simulink model "contrast_stretch_color"  (R2022a)
settings: Solver=FixedStepDiscrete  StartTime=0.0  StopTime=Ts_240p*20  RelTol=1e-3
InitFcn:
  | Ts = 1e-3;
  | Ts_240p = 402*324*Ts;
  | Ts_480p = 525*800*Ts;
undefined symbols (not defined in the file or in its folder): gray, Rec, SDTV
libraries: hdlsllib x8, visionhdlconversions x2, visionhdlio x2, visionconversions x1, visionanalysis x1, dspvision x1
settings Model: DataTypeOverride=Off  ModifiedByFormat=The MathWorks Inc.  NumberOfSteps=10  Creator=The MathWorks, Inc.  LastModifiedBy=The MathWorks Inc.
settings SolverCC: AlgebraicLoopSolver=TrustRegion
settings DataIOCC: LimitDataPoints=on  SaveFormat=Array  SaveOutput=off  SaveTime=off  ReturnWorkspaceOutputs=off
settings OptimizationCC: BlockReduction=off  ConditionallyExecuteInputs=off  DefaultParameterBehavior=Inlined  LifeSpan=inf
settings DebuggingCC: AlgebraicLoopMsg=error  SolverPrmCheckMsg=warning  SingleTaskRateTransMsg=error  ParameterPrecisionLossMsg=none  UnconnectedInputMsg=warning  UnconnectedOutputMsg=warning  UnconnectedLineMsg=warning  AllowSymbolicDim=off  SFUnexpectedBacktrackingDiag=warning  SFNoUnconditionalDefaultTransitionDiag=warning  SFExecutionAtInitializationDiag=none  SFMachineParentedDataDiag=warning  IntegerSaturationMsg=none  ArithmeticOperatorsInVariantConditions=warning
settings HardwareCC: ProdBitPerPointer=32  ProdBitPerSizeT=32  ProdBitPerPtrDiffT=32  ProdLargestAtomicFloat=None  ProdIntDivRoundTo=Undefined  ProdEndianess=Unspecified  ProdWordSize=32  ProdHWDeviceType=ASIC/FPGA->ASIC/FPGA  ProdEqTarget=off
settings ModelReferenceCC: PropagateSignalLabelsOutOfModel=off
settings SFSimCC: SimUseLocalCustomCode=off  CustomCodeUndefinedFunction=UseInterfaceOnly
settings RTWCC: RTWUseLocalCustomCode=off  DLArmComputeVersion=19.05
settings CodeAppCC: StateflowObjectComments=on
settings GRTTargetCC: TargetLangStandard=C89/C90 (ANSI)
settings ConfigComp: CovMetricSettings=dw  CovSaveCumulativeToWorkspaceVar=on  CovSaveSingleToWorkspaceVar=on  CovExternalEMLEnable=off  CovSFcnEnable=off

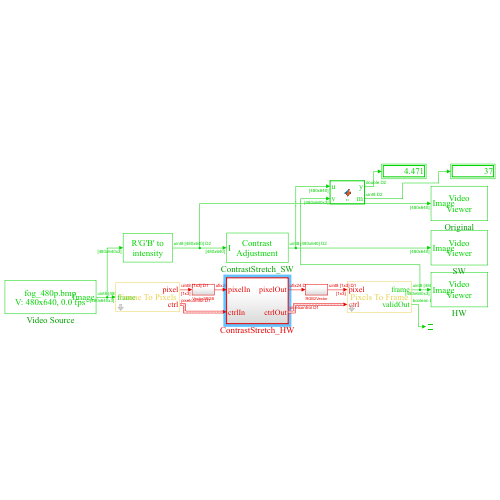
[thumbnail: Simulink's stored preview of the top-level diagram]
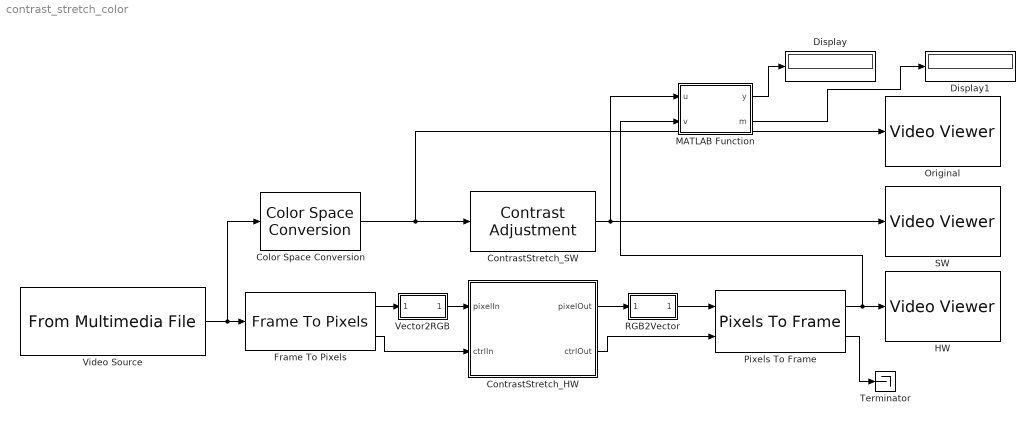
== system contrast_stretch_color ==
  Color Space Conversion : visionconversions/Color Space  Conversion  conversion=Obsolete  conversionActive=R'G'B' to intensity  wp_str=D65  rec=Rec. 601 (SDTV)  sys=1125/60/2:1  imagePorts=One multidimensional signal
  ContrastStretch_HW : Subsystem  TreatAsAtomicUnit=on
  ContrastStretch_SW : visionanalysis/Contrast Adjustment  methodInputRange=Range determined by saturating outlier pixels  rangeIn=[0 73]  fracSaturate=[0.15 0.15]  isBinNum=on  binNum=256  methodOutputRange=Full data type range  rangeOut=[0 255]  roundingMode=Floor  overflowMode=off  prod1Mode=Binary point scaling  prod1WordLength=32  prod1FracLength=16  prod2Mode=Binary point scaling  prod2WordLength=32  prod2FracLength=16
      settings: SourceProductBaseCode=VP
  Display : Display
  Display1 : Display
  Frame To Pixels : visionhdlio/Frame To Pixels  NumComponents=3  NumPixels=1  VideoFormat=480p  ActivePixelsPerLine=640  ActiveVideoLines=480  TotalPixelsPerLine=800  TotalVideoLines=525  StartingActiveLine=36  FrontPorch=16  SampleTime=0  VideoFormatCache=480p  ActivePixelsPerLineCache=32  ActiveVideoLinesCache=18  TotalPixelsPerLineCache=42  TotalVideoLinesCache=28  StartingActiveLineCache=6  FrontPorchCache=5
      settings: SourceProductBaseCode=VT
  HW : VideoViewer  colormapValue=gray(256)  FigPos=[522 705 688 515]
  MATLAB Function : MATLAB Function  TreatAsAtomicUnit=on
  Original : VideoViewer  colormapValue=gray(256)  FigPos=[870 897 688 510]
  Pixels To Frame : visionhdlio/Pixels To Frame  NumComponents=3  NumPixels=1  VideoFormat=480p  ActivePixelsPerLine=640  ActiveVideoLines=480  TotalPixelsPerLine=800  TotalVideoLines=525  VideoFormatCache=480p  ActivePixelsPerLineCache=32  ActiveVideoLinesCache=18  TotalPixelsPerLineCache=42  TotalVideoLinesCache=28
      settings: SourceProductBaseCode=VT
  RGB2Vector : Subsystem
  SW : VideoViewer  colormapValue=gray(256)  FigPos=[295 870 688 514]
  Terminator : Terminator
  Vector2RGB : Subsystem
  Video Source : dspvision/From Multimedia File  inputFilename=D:\datasets\test_images\fog_480p.bmp  readRange=[1 Inf]  loop=on  numPlays=inf  outputStreams=Video only  videoDataType=uint8  audioDataType=int16  inheritSampleTime=off  userDefinedSampleTime=Ts_480p  noAudioOutput=off  isIntensityVideo=off  fourcc=RGB  colorVideoFormat=One multidimensional signal  outputEOF=off  dataOrg=Column-major  audioFrameSize=1024  computeAudioFrameSize=off  outSamplingMode=Sample based
  wires:
  Pixels To Frame/2 -> Terminator/1
  Pixels To Frame/1 -> MATLAB Function/2(v), HW/1
  Vector2RGB/1(RGB) -> ContrastStretch_HW/1(pixelIn)
  ContrastStretch_HW/1(pixelOut) -> RGB2Vector/1(RGB)
  Video Source/1 -> Frame To Pixels/1, Color Space Conversion/1
  Frame To Pixels/2 -> ContrastStretch_HW/2(ctrlIn)
  Frame To Pixels/1 -> Vector2RGB/1(RGBVector)
  RGB2Vector/1(RGBVector) -> Pixels To Frame/1
  ContrastStretch_HW/2(ctrlOut) -> Pixels To Frame/2
  ContrastStretch_SW/1 -> MATLAB Function/1(u), SW/1
  Color Space Conversion/1 -> ContrastStretch_SW/1, Original/1
  MATLAB Function/1(y) -> Display/1
  MATLAB Function/2(m) -> Display1/1

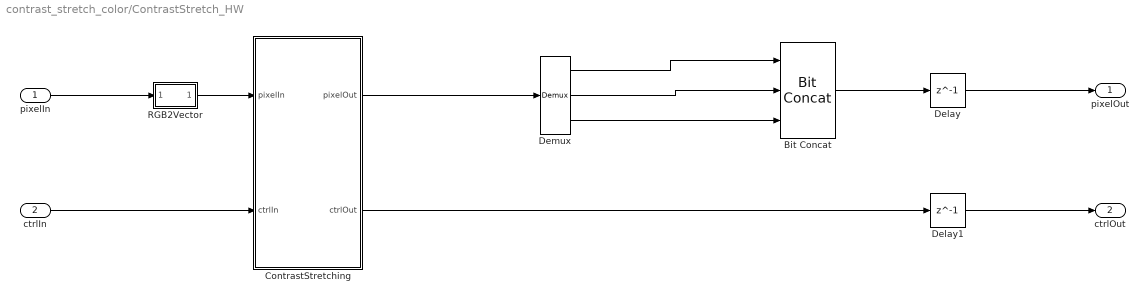
== system contrast_stretch_color/ContrastStretch_HW ==
  pixelIn : Inport
  ctrlIn : Inport  Port=2
  Bit Concat : hdlsllib/Logic and Bit Operations/Bit Concat  numInputs=3
  ContrastStretching : Subsystem  TreatAsAtomicUnit=on
  Delay : Delay  DelayLength=1  InitialCondition=0
  Delay1 : Delay  DelayLength=1  InitialCondition=0
  Demux : Demux  Outputs=3
  RGB2Vector : Subsystem
  pixelOut : Outport  VectorParamsAs1DForOutWhenUnconnected=off
  ctrlOut : Outport  Port=2  VectorParamsAs1DForOutWhenUnconnected=off
  wires:
  ctrlIn/1 -> ContrastStretching/2(ctrlIn)
  pixelIn/1 -> RGB2Vector/1(RGB)
  RGB2Vector/1(RGBVector) -> ContrastStretching/1(pixelIn)
  Bit Concat/1 -> Delay/1
  ContrastStretching/2(ctrlOut) -> Delay1/1
  ContrastStretching/1(pixelOut) -> Demux/1
  Demux/1 -> Bit Concat/1
  Demux/2 -> Bit Concat/2
  Demux/3 -> Bit Concat/3
  Delay/1 -> pixelOut/1
  Delay1/1 -> ctrlOut/1

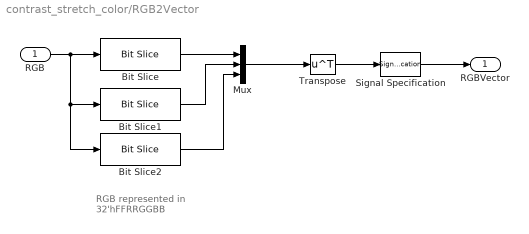
== system contrast_stretch_color/RGB2Vector ==
  note: RGB represented in
      | 32'hFFRRGGBB
  RGB : Inport
  Bit Slice : hdlsllib/Logic and Bit Operations/Bit Slice  lidx=23  ridx=16
      settings: SourceProductBaseCode=SL
  Bit Slice1 : hdlsllib/Logic and Bit Operations/Bit Slice  lidx=15  ridx=8
      settings: SourceProductBaseCode=SL
  Bit Slice2 : hdlsllib/Logic and Bit Operations/Bit Slice  lidx=7  ridx=0
      settings: SourceProductBaseCode=SL
  Mux : Mux  Inputs=3
  Signal Specification : SignalSpecification
  Transpose : Math  Operator=transpose  SignedPower=on
  RGBVector : Outport  VectorParamsAs1DForOutWhenUnconnected=off
  wires:
  Mux/1 -> Transpose/1
  Bit Slice/1 -> Mux/1
  Bit Slice2/1 -> Mux/3
  Bit Slice1/1 -> Mux/2
  RGB/1 -> Bit Slice2/1, Bit Slice1/1, Bit Slice/1
  Transpose/1 -> Signal Specification/1
  Signal Specification/1 -> RGBVector/1

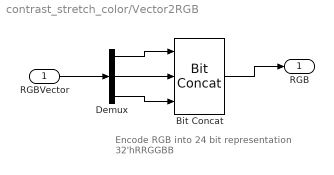
== system contrast_stretch_color/Vector2RGB ==
  note: Encode RGB into 24 bit representation
      | 32'hRRGGBB
  RGBVector : Inport
  Bit Concat : hdlsllib/Logic and Bit Operations/Bit Concat  numInputs=3
  Demux : Demux  Outputs=3
  RGB : Outport  VectorParamsAs1DForOutWhenUnconnected=off
  wires:
  Bit Concat/1 -> RGB/1
  RGBVector/1 -> Demux/1
  Demux/1 -> Bit Concat/1
  Demux/2 -> Bit Concat/2
  Demux/3 -> Bit Concat/3

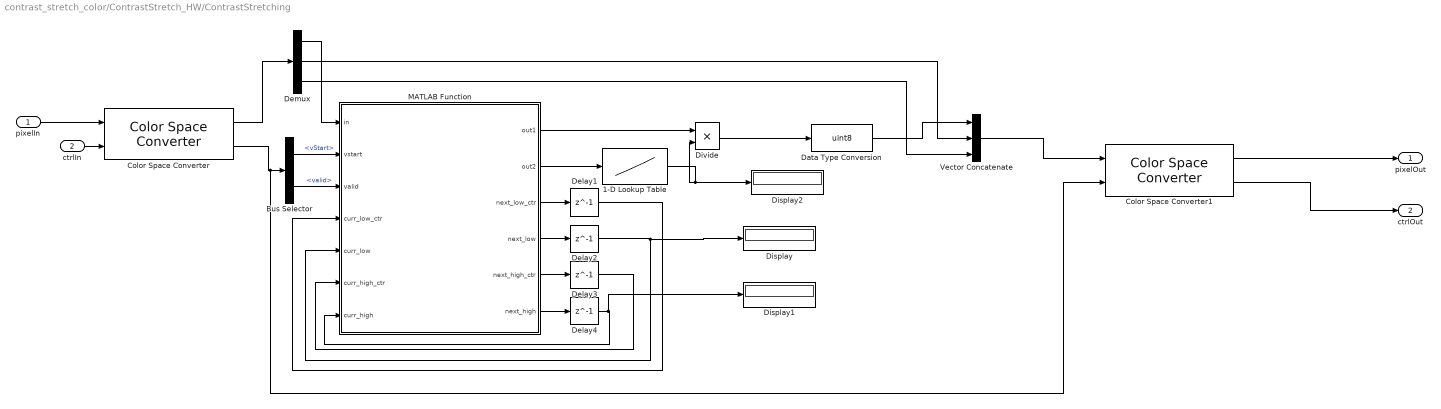
== system contrast_stretch_color/ContrastStretch_HW/ContrastStretching ==
  pixelIn : Inport
  ctrlIn : Inport  Port=2
  1-D Lookup Table : Lookup_n-D  NumberOfTableDimensions=1  LookupTableObject=''  BreakpointsForDimension1=[1:255]  BreakpointsForDimension1FirstPoint=10  BreakpointsForDimension2FirstPoint=10  BreakpointsForDimension1Spacing=12  BreakpointsForDimension2Spacing=12  IndexSearchMethod=Evenly spaced points  Table=1./[1:255]  TableDataTypeStr=fixdt(1,16,15)  InterpMethod=Flat  DiagnosticForOutOfRangeInput=Error  InternalRulePriority=Speed  OutDataTypeStr=fixdt(1,16,15)  RndMeth=Simplest
  Bus Selector : BusSelector  OutputSignals=vStart,valid
  Color Space Converter : visionhdlconversions/Color Space Converter  Conversion=RGB to YCbCr  ConversionStandard=Rec. 601 (SDTV)  ScanningStandard=1250/50/2:1  SimulateUsing=Code generation
      settings: SourceProductBaseCode=VT
  Color Space Converter1 : visionhdlconversions/Color Space Converter  Conversion=YCbCr to RGB  ConversionStandard=Rec. 601 (SDTV)  ScanningStandard=1250/50/2:1  SimulateUsing=Code generation
      settings: SourceProductBaseCode=VT
  Data Type Conversion : DataTypeConversion  OutDataTypeStr=uint8  RndMeth=Floor
  Delay1 : Delay  DelayLength=1  InitialCondition=0
  Delay2 : Delay  DelayLength=1  InitialCondition=100
  Delay3 : Delay  DelayLength=1  InitialCondition=0
  Delay4 : Delay  DelayLength=1  InitialCondition=132
  Demux : Demux  Outputs=3
  Display : Display
  Display1 : Display
  Display2 : Display
  Divide : Product  Inputs=**  RndMeth=Zero
  MATLAB Function : MATLAB Function  TreatAsAtomicUnit=on
  Vector Concatenate : Concatenate  NumInputs=3  Mode=Multidimensional array  ConcatenateDimension=2
  pixelOut : Outport  VectorParamsAs1DForOutWhenUnconnected=off
  ctrlOut : Outport  Port=2  VectorParamsAs1DForOutWhenUnconnected=off
  wires:
  pixelIn/1 -> Color Space Converter/1
  ctrlIn/1 -> Color Space Converter/2
  Color Space Converter/2 -> Color Space Converter1/2, Bus Selector/1
  MATLAB Function/3(next_low_ctr) -> Delay1/1
  Delay1/1 -> MATLAB Function/4(curr_low_ctr)
  MATLAB Function/4(next_low) -> Delay2/1
  Delay2/1 -> Display/1, MATLAB Function/5(curr_low)
  Bus Selector/1 -> MATLAB Function/2(vstart)  "<vStart>"
  Bus Selector/2 -> MATLAB Function/3(valid)  "<valid>"
  MATLAB Function/5(next_high_ctr) -> Delay3/1
  MATLAB Function/6(next_high) -> Delay4/1
  Delay4/1 -> Display1/1, MATLAB Function/7(curr_high)
  Delay3/1 -> MATLAB Function/6(curr_high_ctr)
  MATLAB Function/2(out2) -> 1-D Lookup Table/1
  MATLAB Function/1(out1) -> Divide/1
  1-D Lookup Table/1 -> Display2/1, Divide/2
  Data Type Conversion/1 -> Vector Concatenate/1
  Divide/1 -> Data Type Conversion/1
  Color Space Converter/1 -> Demux/1
  Demux/1 -> MATLAB Function/1(in)
  Demux/3 -> Vector Concatenate/3
  Vector Concatenate/1 -> Color Space Converter1/1
  Color Space Converter1/1 -> pixelOut/1
  Color Space Converter1/2 -> ctrlOut/1
  Demux/2 -> Vector Concatenate/2

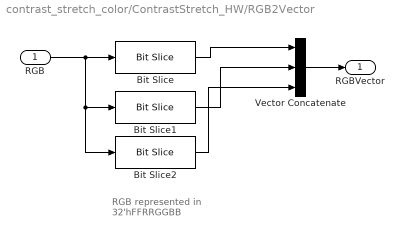
== system contrast_stretch_color/ContrastStretch_HW/RGB2Vector ==
  note: RGB represented in
      | 32'hFFRRGGBB
  RGB : Inport
  Bit Slice : hdlsllib/Logic and Bit Operations/Bit Slice  lidx=23  ridx=16
      settings: SourceProductBaseCode=SL
  Bit Slice1 : hdlsllib/Logic and Bit Operations/Bit Slice  lidx=15  ridx=8
      settings: SourceProductBaseCode=SL
  Bit Slice2 : hdlsllib/Logic and Bit Operations/Bit Slice  lidx=7  ridx=0
      settings: SourceProductBaseCode=SL
  Vector Concatenate : Concatenate  NumInputs=3  Mode=Multidimensional array  ConcatenateDimension=2
  RGBVector : Outport  VectorParamsAs1DForOutWhenUnconnected=off
  wires:
  Bit Slice/1 -> Vector Concatenate/1
  Bit Slice2/1 -> Vector Concatenate/3
  Bit Slice1/1 -> Vector Concatenate/2
  RGB/1 -> Bit Slice2/1, Bit Slice1/1, Bit Slice/1
  Vector Concatenate/1 -> RGBVector/1

== matlab function contrast_stretch_color/MATLAB Function ==
  data: u input; y output; v input; m output
function [y,m] = fcn(u,v)
v = v(:,:,1);
s = size(v);
y = sum(sum(abs(u-v)))/(s(1)*s(2));
m = max(max(abs(u-v)));

== matlab function contrast_stretch_color/ContrastStretch_HW/ContrastStretching/MATLAB Function ==
  data: in input; vstart input; valid input; out1 output fixdt(0,16,0) size=[1,1]; out2 output fixdt(0,8,0) size=[1,1]; curr_low_ctr input fixdt(0,20,0) size=1; next_low_ctr output fixdt(0,20,0) size=1; curr_low input fixdt(0,8,0) size=1; next_low output fixdt(0,8,0) size=1; curr_high_ctr input fixdt(0,20,0) size=1; curr_high input fixdt(0,8,0) size=1; next_high_ctr output fixdt(0,20,0) size=1; next_high output fixdt(0,8,0) size=1
function [out1, out2, next_low_ctr, next_low, next_high_ctr, next_high] = calc_limits(in, vstart, valid, curr_low_ctr, curr_low, curr_high_ctr, curr_high)

% fi(v,s,w,F) returns a fixed-point object with value v, signed property value s, wordlength w, best precision fraction-length and 
%       embedded.fimath F.
      
prob_limit = 2*(640*480)/100;
step = 1;

if(vstart==1)
    next_low_ctr = fi(0,0,20,0);
else
    if((in<curr_low)&(valid==1))
        next_low_ctr = fi(curr_low_ctr + 1,0,20,0);
    else
        next_low_ctr = curr_low_ctr;
    end
end

if(vstart==1)
    if(curr_low_ctr<=prob_limit)%150*curr_low)
        next_low = fi(curr_low + step,0,8,0);
    else
%         if(curr_low>0)
            next_low = fi(curr_low - step,0,8,0);
%         else
%             next_low = curr_low;
%         end
    end
else
    next_low = curr_low;
end

if(vstart==1)
    next_high_ctr = fi(0,0,20,0);
else
    if((in>curr_high)&(valid==1))
        next_high_ctr = fi(curr_high_ctr + 1,0,20,0);
    else
        next_high_ctr = curr_high_ctr;
    end
end

if(vstart==1)
    if(curr_high_ctr<=prob_limit)%150*(255-curr_high))
        next_high = fi(curr_high - step,0,8,0);
    else
%         if(curr_low>0)
            next_high = fi(curr_high + step,0,8,0);
%         else
%             next_low = curr_low;
%         end
    end
else
    next_high = curr_high;
end


low = curr_low;
high = curr_high;
out1 = fi(abs(in-low)*255,0,16,0);
out2 = fi((high-low),0,8,0);
